simulink model "Control_Generico_Aumento_Tipo"  (R2016a)
settings: Solver=VariableStepAuto  StartTime=0.0  StopTime=10.0  RelTol=1e-3
values from neighbouring files (symbols this model uses):
  A = flip(fliplr(A))    [Parcial2024.m]
  B = flip(B)    [Parcial2024.m]
  C = fliplr(C)    [Parcial2024.m]
  Init_cond = 0    [Parcial2024.m]
undefined symbols (not defined in the file or in its folder): D, Kr
settings Model: Creator=adrie  LastModifiedBy=adrie
settings GRTTargetCC: GeneratePreprocessorConditionals=Use local settings

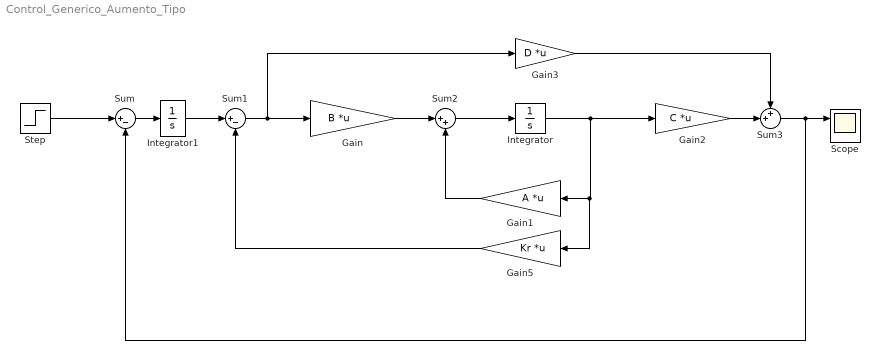
== system Control_Generico_Aumento_Tipo ==
  Gain : Gain  Gain=B  Multiplication=Matrix(K*u) (u vector)
  Gain1 : Gain  Gain=A  Multiplication=Matrix(K*u) (u vector)
  Gain2 : Gain  Gain=C  Multiplication=Matrix(K*u) (u vector)
  Gain3 : Gain  Gain=D  Multiplication=Matrix(K*u) (u vector)
  Gain5 : Gain  Gain=Kr  Multiplication=Matrix(K*u) (u vector)
  Integrator : Integrator  InitialCondition=Init_cond
  Integrator1 : Integrator
  Scope : Scope  NumInputPorts=2
  Step : Step  SampleTime=0
  Sum : Sum  Inputs=|+-
  Sum1 : Sum  Inputs=|+-
  Sum2 : Sum  Inputs=|++
  Sum3 : Sum  Inputs=++|
  wires:
  Gain/1 -> Sum2/1
  Sum2/1 -> Integrator/1
  Gain1/1 -> Sum2/2
  Integrator/1 -> Gain2/1, Gain5/1, Gain1/1
  Gain2/1 -> Sum3/2
  Gain3/1 -> Sum3/1
  Sum3/1 -> Sum/2, Scope/1
  Step/1 -> Sum/1
  Sum/1 -> Integrator1/1
  Gain5/1 -> Sum1/2
  Integrator1/1 -> Sum1/1
  Sum1/1 -> Gain3/1, Gain/1
